simulink model "LoadTest"  (R2016a)
settings: Solver=VariableStepAuto  StartTime=0.0  StopTime=10.0  RelTol=1e-3
undefined symbols (not defined in the file): rad, s
libraries: powerlib x5, aerolibconvert2 x2
settings Model: Creator=Umair  LastModifiedBy=Umair

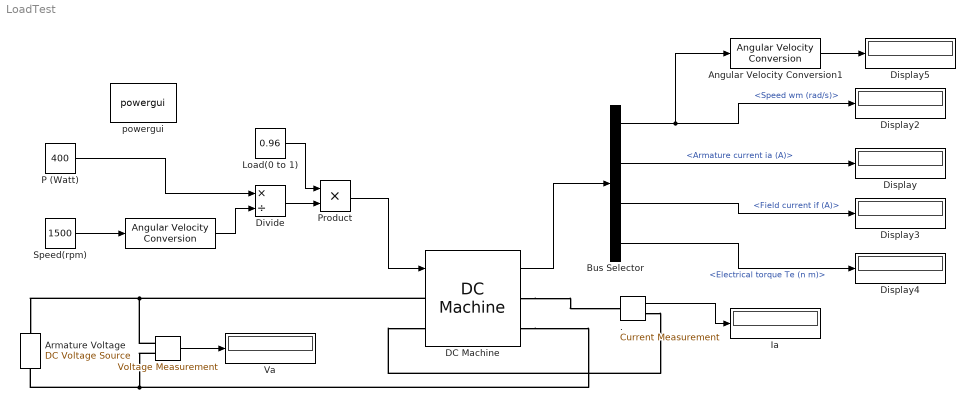
== system LoadTest ==
  " " : powerlib/Measurements/Voltage Measurement  PhasorSimulation=off  OutputType=Complex  PSBequivalent=0
  " " : aerolibconvert2/Angular Velocity Conversion  IU=rpm  OU=rad/s
  . : powerlib/Measurements/Current Measurement  PhasorSimulation=off  OutputType=Complex  PSBequivalent=0
  Angular Velocity Conversion1 : aerolibconvert2/Angular Velocity Conversion  IU=rad/s  OU=rpm
  Armature Voltage : powerlib/Electrical Sources/DC Voltage Source  Amplitude=181.5  Measurements=None
  Bus Selector : BusSelector  OutputSignals=Speed wm (rad/s),Armature current ia (A),Field current if (A),Electrical torque Te (n m)
  DC Machine : powerlib/Machines/DC Machine  PresetModel=No  MechanicalLoad=Torque TL  FieldType=Wound  ShowDetailedParameters=on  MeasurementBus=off  RLa="[ 8  0.016]"  RLf=[ 0.8 122.5]  Laf=1.55  MachineConstant=Torque constant (N.m/A)  Ke=1.8  Kt=1.8  J=0.05  Bm=0.01  Tf=0  w0=0  Ifinit=0  TsPowergui=0  TsBlock=-1
  Display{,2..5} (5 alike) : Display
  Divide : Product  Inputs=*/
  Ia : Display
  Load(0 to 1) : Constant  Value=0.96
  P (Watt) : Constant  Value=400
  Product : Product
  Speed(rpm) : Constant  Value=1500
  Va : Display
  powergui : powerlib/powergui  Priority=1  SimulationMode=Continuous  SolverType=Tustin/Backward Euler (TBE)  SampleTime=50e-6  frequency=60  SPID=off  DisableSnubberDevices=off  DisableRonSwitches=off  DisableVfSwitches=off  SwTol=0  DisplayEquations=off  Interpol=off  ExternalGateDelay=off  methode=off  Ts=10  FunctionMessages=off  echomessages=off  HookPort=off  EnableUseOfTLC=off  x0status=blocks  frequencyindice=0  Pbase=100e6  ErrMax=1e-4  Iterations=50  UnitsV=kV  UnitsW=MW  buscounter=0  RestoreLinks=warning  ResistiveCurrentMeasurement=off  Frange=[0:2:500]  Ylog=off  Xlog=on  ShowGrid=off  save=off  variable=ZData  structure=0  ZoomFFT=off  StartTime=0.0  cycles=1  DisplayStyle=1  fundamental=60  FreqAxis=off  MaxFrequency=1000  frequencyindicesteady=1  RmsSteady=1  display=off
  wires:
  " "/1 -> Va/1
  DC Machine/1 -> Bus Selector/1
  Speed(rpm)/1 -> " "/1
  P (Watt)/1 -> Divide/1
  " "/1 -> Divide/2
  Load(0 to 1)/1 -> Product/1
  Divide/1 -> Product/2
  Product/1 -> DC Machine/1
  Bus Selector/1 -> Angular Velocity Conversion1/1, Display2/1  "<Speed wm (rad/s)>"
  Bus Selector/2 -> Display/1  "<Armature current ia (A)>"
  Bus Selector/3 -> Display3/1  "<Field current if (A)>"
  Bus Selector/4 -> Display4/1  "<Electrical torque Te (n m)>"
  ./1 -> Ia/1
  Angular Velocity Conversion1/1 -> Display5/1
  connections:
  " "/LConn1 -- DC Machine/LConn1 -- Armature Voltage/RConn1
  " "/LConn2 -- DC Machine/RConn2 -- Armature Voltage/LConn1
  DC Machine/RConn1 -- ./LConn1
  ./RConn1 -- DC Machine/LConn2
